simulink subsystem "rotation_model"  (R2025b)
settings: Solver=VariableStepAuto  StartTime=0.0  StopTime=10.0  RelTol=1e-3
values from neighbouring files (symbols this model uses):
  g = 9.81    [params.m]    (also in params_1dof.m; params_3dof.m)
  h = 0.044    [params.m]
  J = sum(e(:).^2)    [ident_model_3dof_closed_loop.m]    (also in params.m = diag([J_xx, J_yy, J_zz]))
  m = 1.210    (= 1.21)    [params.m]    (also in params_1dof.m = 1.014; params_3dof.m = 1.014)
settings Model: Creator=schwmaxi  LastModifiedBy=schwmaxi

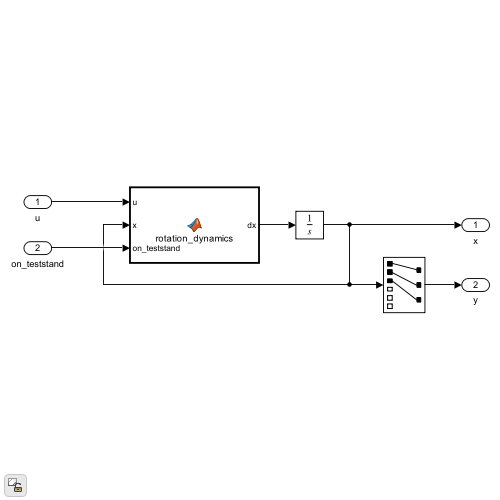
[thumbnail: Simulink's stored preview of the top-level diagram]
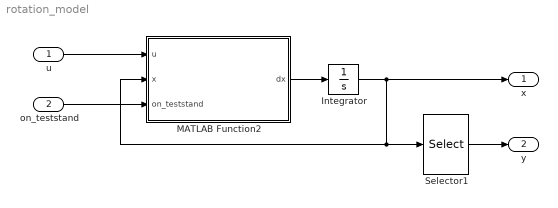
== system rotation_model ==
  u : Inport
  on_teststand : Inport  Port=2
  Integrator : Integrator  InitialCondition=zeros(6, 1)
  MATLAB Function2 : MATLAB Function  TreatAsAtomicUnit=on
  Selector1 : Selector  InputPortWidth=6  IndexOptions=Index vector (dialog)  Indices=[1 2 3]  OutputSizes=1
  x : Outport
  y : Outport  Port=2
  wires:
  u/1 -> MATLAB Function2/1(u)
  on_teststand/1 -> MATLAB Function2/3(on_teststand)
  MATLAB Function2/1(dx) -> Integrator/1
  Selector1/1 -> y/1
  Integrator/1 -> x/1, Selector1/1, MATLAB Function2/2(x)

== matlab function rotation_model/MATLAB Function2 ==
  data: u input; x input; on_teststand input; dx output; J parameter; m parameter; g parameter; h parameter
function dx = rotation_dynamics(u, x, on_teststand, J, m, g, h)
    % J, p, m, g, h  wird als Parameter Data übergeben, vgl. Symbols Pane

    phi = x(1);
    theta = x(2);
    omega = x(4:6);
    
    % transformation matrix
    T = [
        1, sin(phi) * tan(theta), cos(phi)*tan(theta);
        0, cos(phi), -sin(phi);
        0, sin(phi) / cos(theta), cos(phi)/cos(theta);
    ];
    
    tau = u;

    if (on_teststand)
        gravity_moments = [
            m * g * sin(phi) * cos(theta) * h;
            m * g * sin(theta) * h;
            0
        ];
        tau = tau + gravity_moments;
    end

    angles_dot = T * omega;
    omega_dot = J \ (tau - cross(omega, J * omega));

    dx = [angles_dot; omega_dot];
end
